simulink model "EKF_SIL_02_newdelIps"  (R2015a)
settings: Solver=ode45  StartTime=0.0  StopTime=totalSimulationTime  RelTol=1e-3
model workspace: external: MATLAB File Init_Model_02_Simulink_SIL1.m (data not in the file)
values from neighbouring files (symbols this model uses):
  Cov_nu = [0.005 0 0 0 ... (first row only)    [InitOOSM.m]    (also in InitSIL.m; Init_Model_02_Simulink.m; Init_Model_02_Simulink_SIL1.m)
  Cov_r = [0.003 0 0 ... (first row only)    [InitOOSM.m]    (also in InitSIL.m; Init_Model_02_Simulink.m; Init_Model_02_Simulink_SIL1.m)
  e_force_x = 0    [InitOOSM.m]    (also in InitSIL.m; Init_Model_02_Simulink.m; Init_Model_02_Simulink_SIL1.m)
  e_force_y = 0    [InitOOSM.m]    (also in InitSIL.m; Init_Model_02_Simulink.m; Init_Model_02_Simulink_SIL1.m)
  e_force_z = 0    [InitOOSM.m]    (also in InitSIL.m; Init_Model_02_Simulink.m; Init_Model_02_Simulink_SIL1.m)
  ieps = [-0.7071;0;0;0.7071]    [InitOOSM.m]    (also in InitSIL.m; Init_Model_02_Simulink.m = [-0.7071; 0; 0; 0.7071]; Init_Model_02_Simulink_SIL1.m)
  ita = [0.5;0.5;0.5;0.5]    [InitOOSM.m]    (also in InitSIL.m; Init_Model_02_Simulink.m = [0.5; 0.5; 0.5; 0.5]; Init_Model_02_Simulink_SIL1.m)
  n = 0.00    (= 0)    [InitOOSM.m]    (also in InitSIL.m; Init_Model_02_Simulink.m; Init_Model_02_Simulink_SIL1.m)
  P_0 = 0.5*eye(18,18)    [InitOOSM.m]    (also in InitSIL.m = 0.05*eye(12,12); Init_Model_02_Simulink.m = 0.005*eye(12,12); Init_Model_02_Simulink_SIL1.m = 0.005*eye(12,12))
  p_x = 0.75    [InitOOSM.m]    (also in InitSIL.m; Init_Model_02_Simulink.m; Init_Model_02_Simulink_SIL1.m)
  p_y = 0.125    [InitOOSM.m]    (also in InitSIL.m; Init_Model_02_Simulink.m; Init_Model_02_Simulink_SIL1.m)
  p_z = -0.8    [InitOOSM.m]    (also in InitSIL.m; Init_Model_02_Simulink.m; Init_Model_02_Simulink_SIL1.m)
  parameter_gravitation = 3.986005E+14    (= 398600500000000)    [InitOOSM.m]    (also in InitSIL.m; Init_Model_02_Simulink.m; Init_Model_02_Simulink_SIL1.m)
  rho = [0.04;0;0.3]    [InitOOSM.m]    (also in InitSIL.m; Init_Model_02_Simulink.m = [0.04; 0; 0.3]; Init_Model_02_Simulink_SIL1.m)
  rho_c = [-0.00017;   -0.9780;   -0.1854]    [InitOOSM.m]    (also in InitSIL.m = [0.00036;   -0.9865;   -0.1854]; Init_Model_02_Simulink.m = [0.00036; -0.9865; -0.1854]; Init_Model_02_Simulink_SIL1.m = [0.00036;   -0.9865;   -0.1854])
  sig_f = 2E-6    (= 2e-06)    [InitOOSM.m]    (also in InitSIL.m; Init_Model_02_Simulink.m; Init_Model_02_Simulink_SIL1.m)
  sig_tau = 2.5E-5    (= 2.5e-05)    [InitOOSM.m]    (also in InitSIL.m; Init_Model_02_Simulink.m; Init_Model_02_Simulink_SIL1.m)
  t_delta = 0.2    [InitOOSM.m]    (also in InitSIL.m; Init_Model_02_Simulink.m; Init_Model_02_Simulink_SIL1.m)
  t_Kalman = 0.01    [InitOOSM.m]    (also in InitSIL.m; Init_Model_02_Simulink.m; Init_Model_02_Simulink_SIL1.m)
  t_RobotSense = 0.05    [InitOOSM.m]    (also in InitSIL.m; Init_Model_02_Simulink.m; Init_Model_02_Simulink_SIL1.m)
  tau_1 = 0    [InitOOSM.m]    (also in InitSIL.m; Init_Model_02_Simulink.m; Init_Model_02_Simulink_SIL1.m)
  tau_2 = 0    [InitOOSM.m]    (also in InitSIL.m; Init_Model_02_Simulink.m; Init_Model_02_Simulink_SIL1.m)
  tau_3 = 0    [InitOOSM.m]    (also in InitSIL.m; Init_Model_02_Simulink.m; Init_Model_02_Simulink_SIL1.m)
  U_n_d = Simulink.Signal    [InitOOSM.m]    (also in InitSIL.m; Init_Model_02_Simulink.m; Init_Model_02_Simulink_SIL1.m)
  X_a_0 = [0; 0; 0; 1; 0; 0; 0; 0; 0; 0; 0; 0; 0;0;0;0;0;0;0;1]    [InitOOSM.m]    (also in InitSIL.m = [0; 0; 0; 1; 0; 0; 0; 0; 0; 0; 0; 0; 0]; Init_Model_02_Simulink.m = [0;0;0;0.707000000000000;0.707000000000000;0.200000000000000; Init_Model_02_Simulink_SIL1.m = [0;0;0.707;0.707;0.2;-0.02;0.0001;0.02;-1.80;0.50;-0.05;0.00)
libraries: simulink x5, dspmtrx3 x2, aerolibtransform2 x2, visionsinks x1
(part 2 of 4)

== system EKF_SIL_02_newdelIps/EKF/Measurement Update/Create X from X_a ==
  X_a(k) : Inport
  q_nominal(k) : Inport  Port=2
  ieps_nominal : Inport  Port=3
  Bus Creator1 : BusCreator  Inputs=6
  Bus Selector3 : BusSelector  OutputSignals=q_est,omega,r,r_dot,rho_c,ieps
  Bus Selector5 : BusSelector  OutputSignals=q_est,ieps
  Create Bus [State Vector,X_a] : Subsystem
  Create Bus [State Vector] : Subsystem
  Create del_q [body] : Subsystem
  Create del_q [inertial] : Subsystem
  IC : InitialCondition  Value=[X_a_0]
  X(k) : Outport
  q(k) : Outport  Port=2
  ieps(k) : Outport  Port=3
  wires:
  Create Bus [State Vector,X_a]/1(X_bus) -> Bus Selector3/1, Bus Selector5/1
  Create del_q [body]/1(del_q) -> Bus Creator1/1  "del_q"
  Bus Selector3/2 -> Bus Creator1/2  "<omega>"
  Bus Selector3/3 -> Bus Creator1/3  "<r>"
  Bus Selector3/4 -> Bus Creator1/4  "<r_dot>"
  Bus Creator1/1 -> Create Bus [State Vector]/1(X)
  Bus Selector5/1 -> Create del_q [body]/1(q)  "<q_est>"
  Create Bus [State Vector]/1(X_bus) -> X(k)/1
  X_a(k)/1 -> IC/1
  IC/1 -> Create Bus [State Vector,X_a]/1(X)
  Bus Selector3/1 -> q(k)/1  "<q_est>"
  q_nominal(k)/1 -> Create del_q [body]/2(q_nominal)
  ieps_nominal/1 -> Create del_q [inertial]/2(q_nominal)
  Bus Selector5/2 -> Create del_q [inertial]/1(q)  "<ieps>"
  Bus Selector3/5 -> Bus Creator1/5  "<rho_c>"
  Create del_q [inertial]/1(del_q) -> Bus Creator1/6  "del_ieps"
  Bus Selector3/6 -> ieps(k)/1  "<ieps>"

== system EKF_SIL_02_newdelIps/EKF/Measurement Update/Prune P ==
  P_in : Inport
  Constant : Constant  Value=2
  Divide : Product  Inputs=*/
  Math Function : Math  Operator=transpose  SaturateOnIntegerOverflow=on
  Sum : Sum  Inputs=|++
  P_out : Outport
  wires:
  P_in/1 -> Sum/2, Math Function/1
  Math Function/1 -> Sum/1
  Sum/1 -> Divide/1
  Constant/1 -> Divide/2
  Divide/1 -> P_out/1

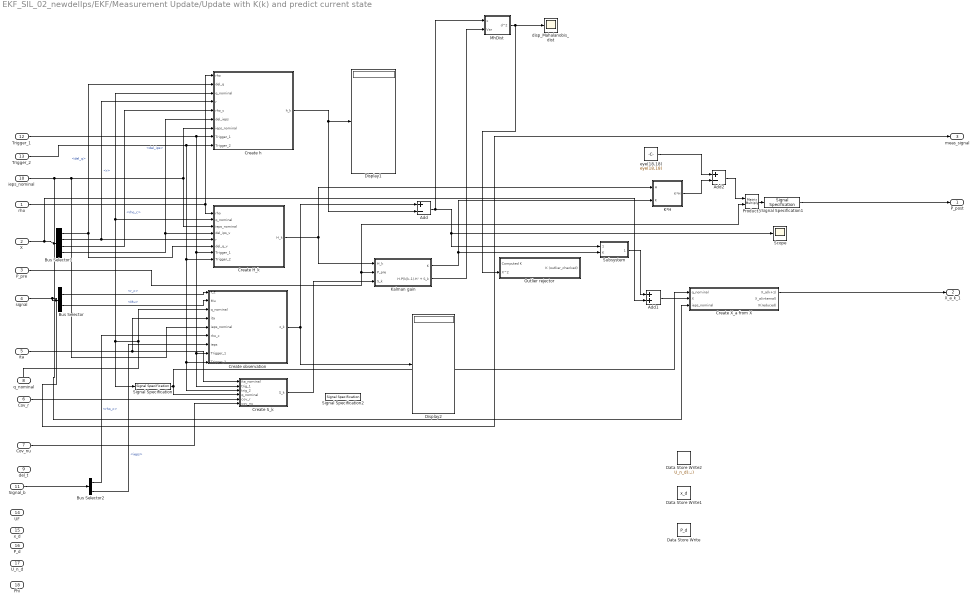
== system EKF_SIL_02_newdelIps/EKF/Measurement Update/Update with K(k) and predict current state ==
  rho : Inport
  X : Inport  Port=2
  P_pre : Inport  Port=3
  signal : Inport  Port=4
  ita : Inport  Port=5
  Cov_r : Inport  Port=6
  Cov_nu : Inport  Port=7
  q_nominal : Inport  Port=8
  del_t : Inport  Port=9
  ieps_nominal : Inport  Port=10
  Signal_b : Inport  Port=11
  Trigger_1 : Inport  Port=12
  Trigger_2 : Inport  Port=13
  UF : Inport  Port=14
  x_d : Inport  Port=15
  P_d : Inport  Port=16
  U_n_d : Inport  Port=17
  Phi : Inport  Port=18
  Add : Sum  Inputs=+-
  Add1 : Sum
  Add2 : Sum  Inputs=+-
  Bus Selector : BusSelector  OutputSignals=r_c,Mu
  Bus Selector1 : BusSelector  OutputSignals=del_q,r,rho_c,del_ips
  Bus Selector2 : BusSelector  OutputSignals=rho_c,ieps
  Create H_k : Subsystem
  Create S_k : Subsystem
  Create X_a from X : Subsystem
  Create h : Subsystem
  Create observation : Subsystem
  Data Store Write : DataStoreWrite  DataStoreName=P_d
  Data Store Write1 : DataStoreWrite  DataStoreName=x_d
  Data Store Write2 : DataStoreWrite  DataStoreName=U_n_d  DataStoreElements=U_n_d(:,:)
  Display1 : Display
  Display2 : Display
  K*H : Subsystem
  Kalman gain : Subsystem
  MhDist : Subsystem
  Outlier rejector : Subsystem
  Product3 : Product  Multiplication=Matrix(*)
  Scope : Scope
      settings: YMin=-0.005  YMax=0.03  SaveName=ScopeData10
  Signal Specification : SignalSpecification  Dimensions=[4,1]
  Signal Specification1 : SignalSpecification  Dimensions=[18,18]
  Signal Specification2 : SignalSpecification  Dimensions=[12,12]
  Subsystem : Subsystem
  disp_Mahalanobis_dist : Scope
      settings: TimeRange=100  YMin=0  YMax=32500  SaveName=ScopeData29
  eye(18,18) : Constant  Value=eye(18,18)
  P_post : Outport
  X_a_k_1 : Outport  Port=2
  meas_signal : Outport  Port=3
  wires:
  Bus Selector/1 -> Create observation/1(r_c)  "<r_c>"
  eye(18,18)/1 -> Add2/1
  Create h/1(h_k) -> Add/2, Display1/1
  Add/1 -> MhDist/1(x), Subsystem/1(residual), Scope/1
  Create observation/1(z_k) -> Add/1, Display2/1
  Bus Selector1/2 -> Create H_k/5(r), Create h/4(r)  "<r>"
  Bus Selector1/1 -> Create h/2(del_q), Create H_k/6(del_q_v)  "<del_q>"
  Create H_k/1(H_k) -> K*H/1(H), Kalman gain/1(H_k)
  P_pre/1 -> Product3/2, Kalman gain/2(P_pre)
  rho/1 -> Create h/1(rho), Create H_k/1(rho)
  Bus Selector/2 -> Create observation/2(Mu)  "<Mu>"
  Add2/1 -> Product3/1
  Signal Specification/1 -> Create S_k/4(q_nominal), Create X_a from X/1(q_nominal)
  Product3/1 -> Signal Specification1/1
  Signal Specification1/1 -> P_post/1
  ita/1 -> Create S_k/1(ita_nominal), Create observation/4(ita)
  signal/1 -> meas_signal/1, Bus Selector/1
  q_nominal/1 -> Signal Specification/1, Create h/3(q_nominal), Create H_k/2(q_nominal), Create observation/3(q_nominal)
  Create X_a from X/1(X_a(k+1)) -> X_a_k_1/1
  Kalman gain/1(K) -> Subsystem/2(K), K*H/2(K)
  Bus Selector1/3 -> Create h/5(rho_c)  "<rho_c>"
  Bus Selector1/4 -> Create h/6("del_ieps "), Create H_k/4(del_ips_v)  "<del_ips>"
  ieps_nominal/1 -> Create X_a from X/3(ieps_nominal), Create observation/5(ieps_nominal), Create H_k/3(ieps_nominal), Create h/7("ieps_nominal ")
  Add1/1 -> Create X_a from X/2(X)
  X/1 -> Add1/2, Bus Selector1/1
  Signal_b/1 -> Bus Selector2/1
  Bus Selector2/1 -> Create observation/6(rho_c)  "<rho_c>"
  Bus Selector2/2 -> Create observation/7(ieps)  "<ieps>"
  Trigger_1/1 -> Create h/8(Trigger_1), Create H_k/7(Trigger_1), Create S_k/2(trig_1), Create observation/8(Trigger_1)
  Trigger_2/1 -> Create h/9(Trigger_2), Create H_k/8(Trigger_2), Create observation/9(Trigger_2), Create S_k/3(trig_2)
  Cov_r/1 -> Create S_k/5(cov_r)
  Cov_nu/1 -> Create S_k/6(cov_nu)
  Create S_k/1(S_k) -> Kalman gain/3(S_k)
  K*H/1(K*H) -> Add2/2
  Subsystem/1(K(z-h(x))) -> Add1/1
  MhDist/1(d^2) -> Outlier rejector/2(X^2), disp_Mahalanobis_dist/1
  Kalman gain/2(H.P(k|k-1).H' + S_k) -> MhDist/2(Var)

== system EKF_SIL_02_newdelIps/EKF/Predictor/Create Bus [State Vector,X_a] ==
  X : Inport
  Bus Creator{1,3..5} (4 alike) : BusCreator  Inputs=3
  Bus Creator2 : BusCreator
  Bus Creator6 : BusCreator  Inputs=6
  Bus Creator7 : BusCreator
  Demux1 : Demux  Outputs=20
  X_bus : Outport
  wires:
  Bus Creator2/1 -> Bus Creator6/1  "q_est"
  Bus Creator3/1 -> Bus Creator6/2  "omega"
  Bus Creator4/1 -> Bus Creator6/3  "r"
  Bus Creator5/1 -> Bus Creator6/4  "r_dot"
  Bus Creator6/1 -> X_bus/1
  X/1 -> Demux1/1
  Demux1/1 -> Bus Creator2/1  "q_est_1"
  Demux1/2 -> Bus Creator2/2  "q_est_2"
  Demux1/3 -> Bus Creator2/3  "q_est_3"
  Demux1/4 -> Bus Creator2/4  "q_est_0"
  Demux1/5 -> Bus Creator3/1  "omega_x"
  Demux1/6 -> Bus Creator3/2  "omega_y"
  Demux1/7 -> Bus Creator3/3  "omega_z"
  Demux1/8 -> Bus Creator4/1  "r_x"
  Demux1/9 -> Bus Creator4/2  "r_y"
  Demux1/10 -> Bus Creator4/3  "r_z"
  Demux1/11 -> Bus Creator5/1  "r_x_dot"
  Demux1/12 -> Bus Creator5/2  "r_y_dot"
  Demux1/13 -> Bus Creator5/3  "r_z_dot"
  Demux1/14 -> Bus Creator1/1  "rho_c_x"
  Demux1/15 -> Bus Creator1/2  "rho_c_y"
  Demux1/16 -> Bus Creator1/3  "rho_c_z"
  Demux1/17 -> Bus Creator7/1  "ieps_1"
  Demux1/18 -> Bus Creator7/2  "ieps_2"
  Demux1/19 -> Bus Creator7/3  "ieps_3"
  Demux1/20 -> Bus Creator7/4  "ieps_0"
  Bus Creator1/1 -> Bus Creator6/5  "rho_c"
  Bus Creator7/1 -> Bus Creator6/6  "ieps"

== system EKF_SIL_02_newdelIps/EKF/Predictor/Create Bus [State Vector,X_a]1 ==
  X : Inport
  Bus Creator{1,3..5} (4 alike) : BusCreator  Inputs=3
  Bus Creator2 : BusCreator
  Bus Creator6 : BusCreator  Inputs=6
  Bus Creator7 : BusCreator
  Demux1 : Demux  Outputs=20
  X_bus : Outport
  wires:
  Bus Creator2/1 -> Bus Creator6/1  "q_est"
  Bus Creator3/1 -> Bus Creator6/2  "omega"
  Bus Creator4/1 -> Bus Creator6/3  "r"
  Bus Creator5/1 -> Bus Creator6/4  "r_dot"
  Bus Creator6/1 -> X_bus/1
  X/1 -> Demux1/1
  Demux1/1 -> Bus Creator2/1  "q_est_1"
  Demux1/2 -> Bus Creator2/2  "q_est_2"
  Demux1/3 -> Bus Creator2/3  "q_est_3"
  Demux1/4 -> Bus Creator2/4  "q_est_0"
  Demux1/5 -> Bus Creator3/1  "omega_x"
  Demux1/6 -> Bus Creator3/2  "omega_y"
  Demux1/7 -> Bus Creator3/3  "omega_z"
  Demux1/8 -> Bus Creator4/1  "r_x"
  Demux1/9 -> Bus Creator4/2  "r_y"
  Demux1/10 -> Bus Creator4/3  "r_z"
  Demux1/11 -> Bus Creator5/1  "r_x_dot"
  Demux1/12 -> Bus Creator5/2  "r_y_dot"
  Demux1/13 -> Bus Creator5/3  "r_z_dot"
  Demux1/14 -> Bus Creator1/1  "rho_c_x"
  Demux1/15 -> Bus Creator1/2  "rho_c_y"
  Demux1/16 -> Bus Creator1/3  "rho_c_z"
  Demux1/17 -> Bus Creator7/1  "ieps_1"
  Demux1/18 -> Bus Creator7/2  "ieps_2"
  Demux1/19 -> Bus Creator7/3  "ieps_3"
  Demux1/20 -> Bus Creator7/4  "ieps_0"
  Bus Creator1/1 -> Bus Creator6/5  "rho_c"
  Bus Creator7/1 -> Bus Creator6/6  "ieps"

== system EKF_SIL_02_newdelIps/EKF/Predictor/Create State error covariance (P) ==
  X_a : Inport
  P_previous : Inport  Port=2
  V : Inport  Port=3
  Add : Sum
  Math Function : Math  Operator=transpose  SaturateOnIntegerOverflow=on
  Matrix Concatenate : Concatenate  NumInputs=3  Mode=Multidimensional array  ConcatenateDimension=2
  Matrix Concatenate1 : Concatenate  NumInputs=3  Mode=Multidimensional array
  Matrix Concatenate2 : Concatenate  NumInputs=3  Mode=Multidimensional array  ConcatenateDimension=2
  Matrix Concatenate3 : Concatenate  NumInputs=3  Mode=Multidimensional array  ConcatenateDimension=2
  "Process Noise [Robot motion] " : Constant  Value=1e-15*eye(6,6)
  Process noise covariance [rotational] : Subsystem
  Process noise covariance [translational] : Subsystem
  Product : Product  Inputs=3  Multiplication=Matrix(*)
  State Propagation : Subsystem
  zeros(6,6) : Constant  Value=zeros(6,6)
  P_current : Outport
  wires:
  Math Function/1 -> Product/3
  P_previous/1 -> Product/2
  Add/1 -> P_current/1
  X_a/1 -> State Propagation/1("X_a(t)\t")
  Product/1 -> Add/2
  Matrix Concatenate2/1 -> Matrix Concatenate1/2
  Matrix Concatenate/1 -> Matrix Concatenate1/1
  zeros(6,6)/1 -> Matrix Concatenate/3, Matrix Concatenate/2, Matrix Concatenate2/3, Matrix Concatenate3/2, Matrix Concatenate3/1, Matrix Concatenate2/1
  State Propagation/1(Phi) -> Math Function/1, Product/1, Process noise covariance [rotational]/1(Phi)
  V/1 -> State Propagation/2(V)
  "Process Noise [Robot motion] "/1 -> Matrix Concatenate3/3
  Matrix Concatenate3/1 -> Matrix Concatenate1/3
  Matrix Concatenate1/1 -> Add/1
  Process noise covariance [rotational]/1(Q_r) -> Matrix Concatenate/1
  Process noise covariance [translational]/1(Q_t) -> Matrix Concatenate2/2

== system EKF_SIL_02_newdelIps/EKF/Predictor/Dynamic Model (Differential equations)2 ==
  X_a(t) : Inport
  "V " : Inport  Port=2
  Dynamic Model (Differential equations) : Subsystem
  X_a_dot : Outport
  wires:
  X_a(t)/1 -> Dynamic Model (Differential equations)/1(X_a(t))
  Dynamic Model (Differential equations)/1(X_a(t+1)) -> X_a_dot/1
  "V "/1 -> Dynamic Model (Differential equations)/2("V ")

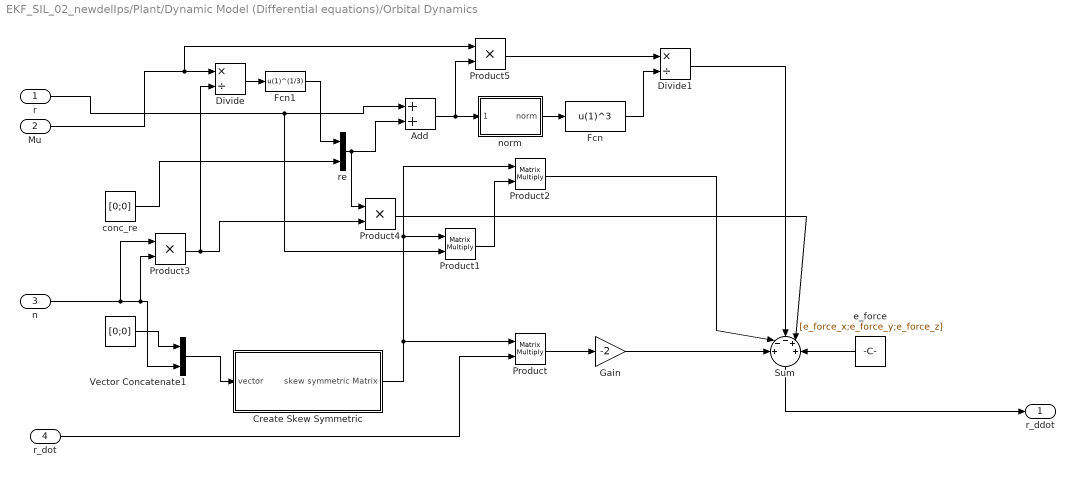
== system EKF_SIL_02_newdelIps/Plant/Dynamic Model (Differential equations)/Orbital Dynamics  ==
  r : Inport
  Mu : Inport  Port=2
  n : Inport  Port=3
  "r_dot " : Inport  Port=4
  " " : Constant  Value=[0;0]
  Add : Sum
  Create Skew Symmetric : Subsystem
  Divide : Product  Inputs=*/
  Divide1 : Product  Inputs=*/
  Fcn : Fcn  Expr=u(1)^3
  Fcn1 : Fcn  Expr=u(1)^(1/3)
  Gain : Gain  Gain=-2
  Product : Product  Multiplication=Matrix(*)
  Product1 : Product  Multiplication=Matrix(*)
  Product2 : Product  Multiplication=Matrix(*)
  Product3 : Product
  Product4 : Product
  Product5 : Product
  Sum : Sum  Inputs=+--++
  Vector Concatenate1 : Concatenate
  "conc_re " : Constant  Value=[0;0]
  "e_force " : Constant  Value=[e_force_x;e_force_y;e_force_z]
  "norm " : Subsystem
  re : Concatenate
  "r_ddot " : Outport
  wires:
  " "/1 -> Vector Concatenate1/1
  Create Skew Symmetric/1(skew symmetric Matrix) -> Product/1, Product1/1, Product2/1
  Product1/1 -> Product2/2
  Mu/1 -> Product5/1, Divide/1
  Product/1 -> Gain/1
  "conc_re "/1 -> re/2
  re/1 -> Product4/1, Add/2
  Product5/1 -> Divide1/1
  "norm "/1("norm ") -> Fcn/1
  n/1 -> Product3/2, Vector Concatenate1/2, Product3/1
  Product3/1 -> Divide/2, Product4/2
  Vector Concatenate1/1 -> Create Skew Symmetric/1(vector)
  Add/1 -> "norm "/1(vector), Product5/2
  Gain/1 -> Sum/1
  Product2/1 -> Sum/2
  r/1 -> Product1/2, Add/1
  Product4/1 -> Sum/4
  "r_dot "/1 -> Product/2
  Divide1/1 -> Sum/3
  Fcn1/1 -> re/1
  Fcn/1 -> Divide1/2
  Divide/1 -> Fcn1/1
  "e_force "/1 -> Sum/5
  Sum/1 -> "r_ddot "/1

== system EKF_SIL_02_newdelIps/Plant/Dynamic Model (Differential equations)/Quaternion Kinematics ==
  q : Inport
  omega_rel : Inport  Port=2
  Constant2 : Constant  Value=0.5
  MATLAB Function : MATLAB Function  TreatAsAtomicUnit=on
  Product : Product  Multiplication=Matrix(*)
  Product1 : Product
  flag : Constant
  q_dot : Outport
  wires:
  MATLAB Function/1(CrossTensor) -> Product/1
  flag/1 -> MATLAB Function/2(flag)
  Constant2/1 -> Product1/2
  q/1 -> MATLAB Function/1(q)
  omega_rel/1 -> Product/2
  Product1/1 -> q_dot/1
  Product/1 -> Product1/1

== system EKF_SIL_02_newdelIps/Plant/Dynamic Model (Differential equations)/Rotational Dynamics ==
  omega : Inport
  p : Inport  Port=2
  Add : Sum
  Create  J : Subsystem
  Create Psi : Subsystem
  Product : Product  Multiplication=Matrix(*)
  tau : Constant  Value=[tau_1;tau_2;tau_3]
  omega_dot : Outport
  wires:
  omega/1 -> Create Psi/1("omega ")
  Create Psi/1(Psi) -> Add/1
  Add/1 -> omega_dot/1
  Product/1 -> Add/2
  p/1 -> Create Psi/2(p), Create  J/1(p)
  Create  J/1("J_k ") -> Product/1
  tau/1 -> Product/2

== system EKF_SIL_02_newdelIps/Plots and display/Create Measurements [Pose]1/Create Measurements [Orientation]  ==
  q : Inport
  "ita " : Inport  Port=2
  Bus Creator : BusCreator
  Demux : Demux
  MATLAB Function : MATLAB Function  TreatAsAtomicUnit=on
  Product : Product  Multiplication=Matrix(*)
  "flag " : Constant  Value=0
  Mu : Outport
  wires:
  Product/1 -> Demux/1
  q/1 -> Product/2
  Bus Creator/1 -> Mu/1  "Mu"
  "ita "/1 -> MATLAB Function/1(q)
  MATLAB Function/1(CrossTensor) -> Product/1
  "flag "/1 -> MATLAB Function/2(flag)
  Demux/1 -> Bus Creator/1
  Demux/2 -> Bus Creator/2
  Demux/3 -> Bus Creator/3
  Demux/4 -> Bus Creator/4

== system EKF_SIL_02_newdelIps/Plots and display/Create Measurements [Pose]1/Create Measurements [Position] ==
  r : Inport
  q : Inport  Port=2
  rho : Inport  Port=3
  "rho_c " : Inport  Port=4
  Add : Sum  Inputs=+++
  Bus Creator : BusCreator  Inputs=3
  "Create Rotation Matrix " : Subsystem
  Demux : Demux  Outputs=3
  Product : Product  Multiplication=Matrix(*)
  r_c : Outport
  wires:
  Add/1 -> Demux/1
  r/1 -> Add/2
  Bus Creator/1 -> r_c/1  "r_c"
  q/1 -> "Create Rotation Matrix "/1(q)
  "rho_c "/1 -> Add/1
  rho/1 -> Product/2
  "Create Rotation Matrix "/1(R) -> Product/1
  Product/1 -> Add/3
  Demux/1 -> Bus Creator/1  "r_c_x"
  Demux/2 -> Bus Creator/2  "r_c_y"
  Demux/3 -> Bus Creator/3  "r_c_z"

== system EKF_SIL_02_newdelIps/Plots and display/Create Measurements [Pose]2/Create Measurements [Orientation]  ==
  q : Inport
  "ita " : Inport  Port=2
  "ieps " : Inport  Port=3
  Bus Creator : BusCreator
  Demux : Demux
  MATLAB Function : MATLAB Function  TreatAsAtomicUnit=on
  MATLAB Function1 : MATLAB Function  TreatAsAtomicUnit=on
  Product : Product  Multiplication=Matrix(*)
  Product1 : Product  Multiplication=Matrix(*)
  "flag " : Constant  Value=0
  Mu : Outport
  wires:
  Demux/4 -> Bus Creator/4
  Demux/3 -> Bus Creator/3
  Demux/2 -> Bus Creator/2
  Demux/1 -> Bus Creator/1
  "flag "/1 -> MATLAB Function1/2(flag), MATLAB Function/2(flag)
  MATLAB Function/1(CrossTensor) -> Product/1
  "ita "/1 -> MATLAB Function/1(q)
  Bus Creator/1 -> Mu/1  "Mu"
  q/1 -> Product/2
  Product/1 -> MATLAB Function1/1(q)
  MATLAB Function1/1(CrossTensor) -> Product1/1
  "ieps "/1 -> Product1/2
  Product1/1 -> Demux/1

== system EKF_SIL_02_newdelIps/Plots and display/Create Measurements [Pose]2/Create Measurements [Position] ==
  r : Inport
  q : Inport  Port=2
  rho : Inport  Port=3
  "rho_c " : Inport  Port=4
  "ieps " : Inport  Port=5
  Add : Sum
  Add1 : Sum
  Bus Creator : BusCreator  Inputs=3
  "Create Rotation Matrix " : Subsystem
  Create Rotation Matrix 1 : Subsystem
  Demux : Demux  Outputs=3
  Product : Product  Multiplication=Matrix(*)
  Product1 : Product  Multiplication=Matrix(*)
  r_c : Outport
  wires:
  Demux/3 -> Bus Creator/3  "r_c_z"
  Demux/2 -> Bus Creator/2  "r_c_y"
  Demux/1 -> Bus Creator/1  "r_c_x"
  Product/1 -> Add/2
  "Create Rotation Matrix "/1(R) -> Product/1
  rho/1 -> Product/2
  q/1 -> "Create Rotation Matrix "/1(q)
  Bus Creator/1 -> r_c/1  "r_c"
  r/1 -> Add/1
  Create Rotation Matrix 1/1(R) -> Product1/1
  "rho_c "/1 -> Add1/2
  Add1/1 -> Demux/1
  Add/1 -> Product1/2
  "ieps "/1 -> Create Rotation Matrix 1/1(q)
  Product1/1 -> Add1/1

== system EKF_SIL_02_newdelIps/EKF/Measurement Update/Create X from X_a/Create Bus [State Vector,X_a] ==
  X : Inport
  Bus Creator{1,3..5} (4 alike) : BusCreator  Inputs=3
  Bus Creator2 : BusCreator
  Bus Creator6 : BusCreator  Inputs=6
  Bus Creator7 : BusCreator
  Demux1 : Demux  Outputs=20
  X_bus : Outport
  wires:
  Bus Creator2/1 -> Bus Creator6/1  "q_est"
  Bus Creator3/1 -> Bus Creator6/2  "omega"
  Bus Creator4/1 -> Bus Creator6/3  "r"
  Bus Creator5/1 -> Bus Creator6/4  "r_dot"
  Bus Creator6/1 -> X_bus/1
  X/1 -> Demux1/1
  Demux1/1 -> Bus Creator2/1  "q_est_1"
  Demux1/2 -> Bus Creator2/2  "q_est_2"
  Demux1/3 -> Bus Creator2/3  "q_est_3"
  Demux1/4 -> Bus Creator2/4  "q_est_0"
  Demux1/5 -> Bus Creator3/1  "omega_x"
  Demux1/6 -> Bus Creator3/2  "omega_y"
  Demux1/7 -> Bus Creator3/3  "omega_z"
  Demux1/8 -> Bus Creator4/1  "r_x"
  Demux1/9 -> Bus Creator4/2  "r_y"
  Demux1/10 -> Bus Creator4/3  "r_z"
  Demux1/11 -> Bus Creator5/1  "r_x_dot"
  Demux1/12 -> Bus Creator5/2  "r_y_dot"
  Demux1/13 -> Bus Creator5/3  "r_z_dot"
  Demux1/14 -> Bus Creator1/1  "rho_c_x"
  Demux1/15 -> Bus Creator1/2  "rho_c_y"
  Demux1/16 -> Bus Creator1/3  "rho_c_z"
  Demux1/17 -> Bus Creator7/1  "ieps_1"
  Demux1/18 -> Bus Creator7/2  "ieps_2"
  Demux1/19 -> Bus Creator7/3  "ieps_3"
  Demux1/20 -> Bus Creator7/4  "ieps_0"
  Bus Creator1/1 -> Bus Creator6/5  "rho_c"
  Bus Creator7/1 -> Bus Creator6/6  "ieps"

== system EKF_SIL_02_newdelIps/EKF/Measurement Update/Create X from X_a/Create Bus [State Vector] ==
  X : Inport
  Bus Creator{1..5,7} (6 alike) : BusCreator  Inputs=3
  Bus Creator6 : BusCreator  Inputs=6
  Demux1 : Demux  Outputs=18
  X_bus : Outport
  wires:
  Demux1/4 -> Bus Creator3/1  "omega_x"
  Bus Creator2/1 -> Bus Creator6/1  "del_q"
  Demux1/8 -> Bus Creator4/2  "r_y"
  Demux1/6 -> Bus Creator3/3  "omega_z"
  Demux1/7 -> Bus Creator4/1  "r_x"
  Demux1/10 -> Bus Creator5/1  "r_x_dot"
  Bus Creator3/1 -> Bus Creator6/2  "omega"
  Demux1/3 -> Bus Creator2/3  "del_q_3"
  Demux1/1 -> Bus Creator2/1  "del_q_1"
  Demux1/11 -> Bus Creator5/2  "r_y_dot"
  Demux1/12 -> Bus Creator5/3  "r_z_dot"
  Demux1/2 -> Bus Creator2/2  "del_q_2"
  Demux1/5 -> Bus Creator3/2  "omega_y"
  Demux1/9 -> Bus Creator4/3  "r_z"
  Bus Creator4/1 -> Bus Creator6/3  "r"
  Bus Creator5/1 -> Bus Creator6/4  "r_dot"
  Bus Creator6/1 -> X_bus/1
  X/1 -> Demux1/1
  Demux1/13 -> Bus Creator1/1  "rho_c_x"
  Demux1/14 -> Bus Creator1/2  "rho_c_y"
  Demux1/15 -> Bus Creator1/3  "rho_c_z"
  Demux1/16 -> Bus Creator7/1  "del_ieps_1"
  Demux1/17 -> Bus Creator7/2
  Demux1/18 -> Bus Creator7/3  "del_ips_3"
  Bus Creator1/1 -> Bus Creator6/5  "rho_c"
  Bus Creator7/1 -> Bus Creator6/6  "del_ips"

== system EKF_SIL_02_newdelIps/EKF/Measurement Update/Create X from X_a/Create del_q [body] ==
  q : Inport
  q_nominal : Inport  Port=2
  Constant : Constant  Value=0
  Demux : Demux
  MATLAB Function : MATLAB Function  TreatAsAtomicUnit=on
  Mux : Mux  Inputs=3
  Product : Product  Multiplication=Matrix(*)
  Scope : Scope
      settings: SaveName=ScopeData6
  q_star : Subsystem
  del_q : Outport
  wires:
  q_star/1(q_star) -> Product/2
  MATLAB Function/1(CrossTensor) -> Product/1
  q/1 -> MATLAB Function/1(q)
  Constant/1 -> MATLAB Function/2(flag)
  q_nominal/1 -> q_star/1(q)
  Product/1 -> Demux/1
  Demux/1 -> Mux/1
  Demux/2 -> Mux/2
  Demux/3 -> Mux/3
  Mux/1 -> del_q/1
  Demux/4 -> Scope/1

== system EKF_SIL_02_newdelIps/EKF/Measurement Update/Create X from X_a/Create del_q [inertial] ==
  q : Inport
  q_nominal : Inport  Port=2
  Constant : Constant  Value=0
  Demux : Demux
  MATLAB Function : MATLAB Function  TreatAsAtomicUnit=on
  Mux : Mux  Inputs=3
  Product : Product  Multiplication=Matrix(*)
  Scope : Scope
      settings: SaveName=ScopeData6
  q_star : Subsystem
  del_q : Outport
  wires:
  q_star/1(q_star) -> Product/2
  MATLAB Function/1(CrossTensor) -> Product/1
  q/1 -> MATLAB Function/1(q)
  Constant/1 -> MATLAB Function/2(flag)
  q_nominal/1 -> q_star/1(q)
  Product/1 -> Demux/1
  Demux/1 -> Mux/1
  Demux/2 -> Mux/2
  Demux/3 -> Mux/3
  Mux/1 -> del_q/1
  Demux/4 -> Scope/1

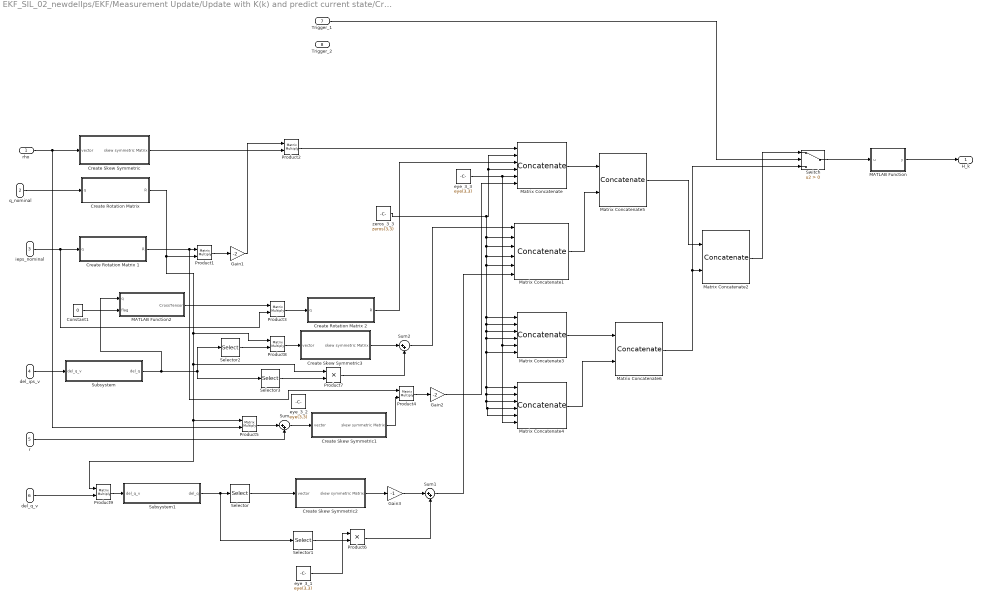
== system EKF_SIL_02_newdelIps/EKF/Measurement Update/Update with K(k) and predict current state/Create H_k ==
  rho : Inport
  q_nominal : Inport  Port=2
  ieps_nominal : Inport  Port=3
  del_ips_v : Inport  Port=4
  r : Inport  Port=5
  del_q_v : Inport  Port=6
  Trigger_1 : Inport  Port=7
  Trigger_2 : Inport  Port=8
  Constant1 : Constant  Value=0
  "Create Rotation Matrix " : Subsystem
  Create Rotation Matrix 1 : Subsystem
  Create Rotation Matrix 2 : Subsystem
  Create Skew Symmetric : Subsystem
  Create Skew Symmetric1 : Subsystem
  Create Skew Symmetric2 : Subsystem
  Create Skew Symmetric3 : Subsystem
  Gain1 : Gain  Gain=-2
  Gain2 : Gain  Gain=-2
  Gain3 : Gain  Gain=-1
  MATLAB Function : MATLAB Function  TreatAsAtomicUnit=on
  MATLAB Function2 : MATLAB Function  TreatAsAtomicUnit=on
  Matrix Concatenate{,1,3..4} (4 alike) : Concatenate  NumInputs=6  Mode=Multidimensional array  ConcatenateDimension=2
  Matrix Concatenate2 : Concatenate  Mode=Multidimensional array
  Matrix Concatenate5 : Concatenate  Mode=Multidimensional array
  Matrix Concatenate6 : Concatenate  Mode=Multidimensional array
  Product{1..5,8..9} (7 alike) : Product  Multiplication=Matrix(*)
  Product6 : Product
  Product7 : Product
  Selector : Selector  InputPortWidth=4  Indices=[1:3]
  Selector1 : Selector  InputPortWidth=4  Indices=4
  Selector2 : Selector  InputPortWidth=4  Indices=[1:3]
  Selector3 : Selector  InputPortWidth=4  Indices=4
  Subsystem : Subsystem
  Subsystem1 : Subsystem
  Sum : Sum  Inputs=|++
  Sum1 : Sum  Inputs=|++
  Sum2 : Sum  Inputs=|++
  Switch : Switch  Criteria=u2 > Threshold  AllowDiffInputSizes=on
  eye_3_1 : Constant  Value=eye(3,3)
  eye_3_2 : Constant  Value=eye(3,3)
  eye_3_3 : Constant  Value=eye(3,3)
  zeros_3_3 : Constant  Value=zeros(3,3)
  H_k : Outport
  wires:
  q_nominal/1 -> "Create Rotation Matrix "/1(q)
  Switch/1 -> MATLAB Function/1(u)
  eye_3_3/1 -> Matrix Concatenate4/6, Matrix Concatenate3/5, Matrix Concatenate/5
  Create Skew Symmetric/1(skew symmetric Matrix) -> Product2/2
  rho/1 -> Product5/2, Create Skew Symmetric/1(vector)
  Create Rotation Matrix 1/1(R) -> Product4/1, Product1/1
  Product1/1 -> Gain1/1
  Gain1/1 -> Product2/1
  Product2/1 -> Matrix Concatenate/1
  del_ips_v/1 -> Subsystem/1(del_q_v)
  Constant1/1 -> MATLAB Function2/2(flag)
  MATLAB Function2/1(CrossTensor) -> Product3/1
  ieps_nominal/1 -> Product3/2, Create Rotation Matrix 1/1(q)
  Create Rotation Matrix 2/1(R) -> Matrix Concatenate/3
  "Create Rotation Matrix "/1(R) -> Product7/1, Product9/1, Product5/1, Product8/1, Product1/2
  Product5/1 -> Sum/1
  r/1 -> Sum/2
  Gain2/1 -> Matrix Concatenate/6
  Subsystem1/1(del_q) -> Selector1/1, Selector/1
  Selector/1 -> Create Skew Symmetric2/1(vector)
  Create Skew Symmetric2/1(skew symmetric Matrix) -> Gain3/1
  Selector1/1 -> Product6/2
  eye_3_1/1 -> Product6/1
  Gain3/1 -> Sum1/1
  Product6/1 -> Sum1/2
  Sum1/1 -> Matrix Concatenate1/6
  Selector2/1 -> Product8/2
  Create Skew Symmetric3/1(skew symmetric Matrix) -> Sum2/1
  Selector3/1 -> Product7/2
  Product7/1 -> Sum2/2
  Sum2/1 -> Matrix Concatenate1/1
  Sum/1 -> Create Skew Symmetric1/1(vector)
  Create Skew Symmetric1/1(skew symmetric Matrix) -> Product4/2
  Product3/1 -> Create Rotation Matrix 2/1(q)
  zeros_3_3/1 -> Matrix Concatenate3/6, Matrix Concatenate4/1, Matrix Concatenate4/5, Matrix Concatenate4/4, Matrix Concatenate4/3, Matrix Concatenate4/2, Matrix Concatenate3/4, Matrix Concatenate3/3, Matrix Concatenate3/2, Matrix Concatenate3/1, Matrix Concatenate1/5, Matrix Concatenate1/4, Matrix Concatenate1/3, Matrix Concatenate1/2, Matrix Concatenate/4, Matrix Concatenate/2
  Matrix Concatenate1/1 -> Matrix Concatenate5/2
  Matrix Concatenate4/1 -> Matrix Concatenate6/2
  Subsystem/1(del_q) -> MATLAB Function2/1(q), Selector2/1, Selector3/1
  del_q_v/1 -> Product9/2
  Product9/1 -> Subsystem1/1(del_q_v)
  Product8/1 -> Create Skew Symmetric3/1(vector)
  Product4/1 -> Gain2/1
  Matrix Concatenate/1 -> Matrix Concatenate5/1
  Matrix Concatenate3/1 -> Matrix Concatenate6/1
  Trigger_1/1 -> Switch/2
  Matrix Concatenate5/1 -> Matrix Concatenate2/1
  Matrix Concatenate6/1 -> Switch/3, Matrix Concatenate2/2
  Matrix Concatenate2/1 -> Switch/1
  MATLAB Function/1(y) -> H_k/1

== system EKF_SIL_02_newdelIps/EKF/Measurement Update/Update with K(k) and predict current state/Create S_k ==
  ita_nominal : Inport
  trig_1 : Inport  Port=2
  trig_2 : Inport  Port=3
  q_nominal : Inport  Port=4
  cov_r : Inport  Port=5
  cov_nu : Inport  Port=6
  Constant : Constant  Value=1e-5*eye(6,6)
  Constant1 : Constant  Value=zeros(6,6)
  Matrix Concatenate1 : Concatenate  Mode=Multidimensional array
  Matrix Concatenate5 : Concatenate  Mode=Multidimensional array  ConcatenateDimension=2
  Matrix Concatenate6 : Concatenate  Mode=Multidimensional array  ConcatenateDimension=2
  Measurement noise covariance : MATLAB Function  TreatAsAtomicUnit=on
  Switch : Switch  Criteria=u2 > Threshold  AllowDiffInputSizes=on
  S_k : Outport
  wires:
  q_nominal/1 -> Measurement noise covariance/1(q_nominal)
  ita_nominal/1 -> Measurement noise covariance/2(ita_nominal)
  cov_nu/1 -> Measurement noise covariance/4(cov_nu)
  cov_r/1 -> Measurement noise covariance/3(cov_r)
  Measurement noise covariance/1(S) -> Matrix Concatenate5/1, Switch/3
  trig_1/1 -> Switch/2
  Constant1/1 -> Matrix Concatenate6/1, Matrix Concatenate5/2
  Constant/1 -> Matrix Concatenate6/2
  Switch/1 -> S_k/1
  Matrix Concatenate1/1 -> Switch/1
  Matrix Concatenate5/1 -> Matrix Concatenate1/1
  Matrix Concatenate6/1 -> Matrix Concatenate1/2

== system EKF_SIL_02_newdelIps/EKF/Measurement Update/Update with K(k) and predict current state/Create X_a from X ==
  q_nominal : Inport
  X : Inport  Port=2
  ieps_nominal : Inport  Port=3
  Bus Creator1 : BusCreator
  Bus Creator2 : BusCreator  Inputs=6
  Bus Creator3 : BusCreator
  Bus Selector2 : BusSelector  OutputSignals=del_q,del_ips
  Bus Selector3 : BusSelector  OutputSignals=omega,r,r_dot,rho_c
  Create Bus [State Vector] : Subsystem
  "Create ieps " : Subsystem
  "Create q_nominal " : Subsystem
  Demux : Demux
  Demux1 : Demux
  Display2 : Display
  Signal Conversion : SignalConversion
  X_a(k+1) : Outport
  X_a(internal) : Outport  Port=2
  "X(reduced) " : Outport  Port=3
  wires:
  Bus Selector3/3 -> Bus Creator2/4  "<r_dot>"
  Demux/1 -> Bus Creator3/1  "q_est_1"
  Bus Selector3/2 -> Bus Creator2/3  "<r>"
  Bus Creator3/1 -> Bus Creator2/1  "q_est"
  Create Bus [State Vector]/1(X_bus) -> "X(reduced) "/1, Bus Selector3/1, Bus Selector2/1
  X/1 -> Create Bus [State Vector]/1(X)
  Bus Selector3/1 -> Bus Creator2/2  "<omega>"
  Demux/2 -> Bus Creator3/2  "q_est_2"
  Demux/4 -> Bus Creator3/4  "q_est_0"
  Demux/3 -> Bus Creator3/3  "q_est_3"
  Bus Creator2/1 -> X_a(internal)/1, Signal Conversion/1
  Bus Selector2/1 -> "Create q_nominal "/1(del_q)  "<del_q>"
  q_nominal/1 -> "Create q_nominal "/2(q_nominal)
  "Create q_nominal "/1(q_est) -> Demux/1
  Signal Conversion/1 -> X_a(k+1)/1
  Bus Selector2/2 -> "Create ieps "/1(del_q)  "<del_ips>"
  ieps_nominal/1 -> "Create ieps "/2(q_nominal)
  Bus Selector3/4 -> Bus Creator2/5  "<rho_c>"
  Demux1/1 -> Bus Creator1/1  "ieps_est_1"
  Bus Creator1/1 -> Bus Creator2/6  "ieps_est"
  Demux1/2 -> Bus Creator1/2  "ieps_est_2"
  Demux1/4 -> Bus Creator1/4  "ieps_est_0"
  Demux1/3 -> Bus Creator1/3  "ieps_est_3"
  "Create ieps "/1(q_est) -> Display2/1, Demux1/1

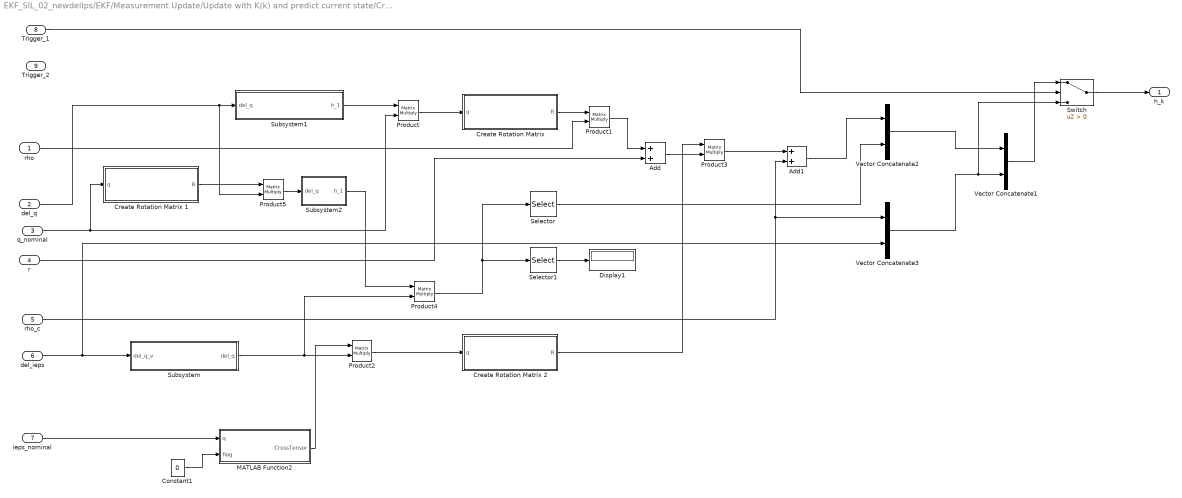
== system EKF_SIL_02_newdelIps/EKF/Measurement Update/Update with K(k) and predict current state/Create h ==
  rho : Inport
  del_q : Inport  Port=2
  q_nominal : Inport  Port=3
  r : Inport  Port=4
  rho_c : Inport  Port=5
  "del_ieps " : Inport  Port=6
  "ieps_nominal " : Inport  Port=7
  Trigger_1 : Inport  Port=8
  Trigger_2 : Inport  Port=9
  Add : Sum
  Add1 : Sum
  Constant1 : Constant  Value=0
  "Create Rotation Matrix " : Subsystem
  Create Rotation Matrix 1 : Subsystem
  Create Rotation Matrix 2 : Subsystem
  Display1 : Display
  MATLAB Function2 : MATLAB Function  TreatAsAtomicUnit=on
  Product{,1..5} (6 alike) : Product  Multiplication=Matrix(*)
  Selector : Selector  InputPortWidth=4  Indices=[1:3]
  Selector1 : Selector  InputPortWidth=4  Indices=4
  Subsystem : Subsystem
  Subsystem1 : Subsystem
  Subsystem2 : Subsystem
  Switch : Switch  Criteria=u2 > Threshold  AllowDiffInputSizes=on
  Vector Concatenate1 : Concatenate
  Vector Concatenate2 : Concatenate
  Vector Concatenate3 : Concatenate
  h_k : Outport
  wires:
  rho/1 -> Product1/2
  q_nominal/1 -> Product/2, Create Rotation Matrix 1/1(q)
  "Create Rotation Matrix "/1(R) -> Product1/1
  del_q/1 -> Product5/2, Subsystem1/1(del_q)
  Product/1 -> "Create Rotation Matrix "/1(q)
  Subsystem1/1(h_1) -> Product/1
  Product1/1 -> Add/1
  rho_c/1 -> Vector Concatenate3/1, Add1/2
  "del_ieps "/1 -> Vector Concatenate3/2, Subsystem/1(del_q_v)
  "ieps_nominal "/1 -> MATLAB Function2/1(q)
  Constant1/1 -> MATLAB Function2/2(flag)
  Subsystem/1(del_q) -> Product4/2, Product2/2
  MATLAB Function2/1(CrossTensor) -> Product2/1
  Product2/1 -> Create Rotation Matrix 2/1(q)
  Create Rotation Matrix 2/1(R) -> Product3/1
  Product3/1 -> Add1/1
  Add/1 -> Product3/2
  Add1/1 -> Vector Concatenate2/1
  Product4/1 -> Selector1/1, Selector/1
  r/1 -> Add/2
  Selector1/1 -> Display1/1
  Create Rotation Matrix 1/1(R) -> Product5/1
  Product5/1 -> Subsystem2/1(del_q)
  Subsystem2/1(h_1) -> Product4/1
  Selector/1 -> Vector Concatenate2/2
  Trigger_1/1 -> Switch/2
  Vector Concatenate2/1 -> Vector Concatenate1/1
  Vector Concatenate3/1 -> Switch/3, Vector Concatenate1/2
  Switch/1 -> h_k/1
  Vector Concatenate1/1 -> Switch/1

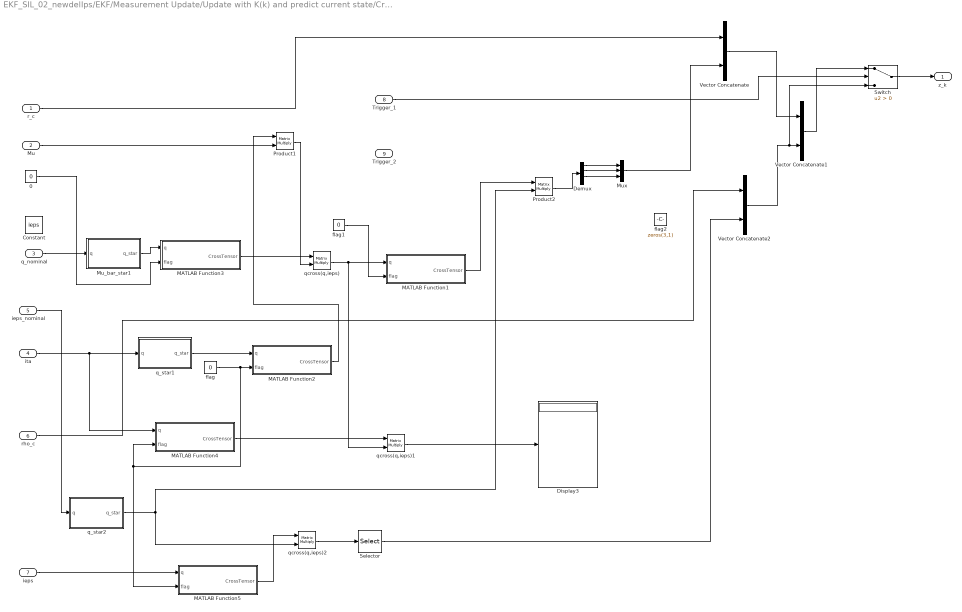
== system EKF_SIL_02_newdelIps/EKF/Measurement Update/Update with K(k) and predict current state/Create observation ==
  r_c : Inport
  Mu : Inport  Port=2
  q_nominal : Inport  Port=3
  ita : Inport  Port=4
  ieps_nominal : Inport  Port=5
  rho_c : Inport  Port=6
  ieps : Inport  Port=7
  Trigger_1 : Inport  Port=8
  Trigger_2 : Inport  Port=9
  0 : Constant  Value=0
  Constant : Constant  Value=ieps
  Demux : Demux
  Display3 : Display
  MATLAB Function1 : MATLAB Function  TreatAsAtomicUnit=on
  MATLAB Function2 : MATLAB Function  TreatAsAtomicUnit=on
  MATLAB Function3 : MATLAB Function  TreatAsAtomicUnit=on
  MATLAB Function4 : MATLAB Function  TreatAsAtomicUnit=on
  MATLAB Function5 : MATLAB Function  TreatAsAtomicUnit=on
  Mu_bar_star1 : Subsystem
  Mux : Mux  Inputs=3
  Product1 : Product  Multiplication=Matrix(*)
  Product2 : Product  Multiplication=Matrix(*)
  Selector : Selector  InputPortWidth=4  Indices=[1:3]
  Switch : Switch  Criteria=u2 > Threshold  AllowDiffInputSizes=on
  Vector Concatenate : Concatenate
  Vector Concatenate1 : Concatenate
  Vector Concatenate2 : Concatenate
  flag : Constant  Value=0
  flag1 : Constant  Value=0
  flag2 : Constant  Value=zeros(3,1)
  q_star1 : Subsystem
  q_star2 : Subsystem
  qcross(q,ieps) : Product  Multiplication=Matrix(*)
  qcross(q,ieps)1 : Product  Multiplication=Matrix(*)
  qcross(q,ieps)2 : Product  Multiplication=Matrix(*)
  z_k : Outport
  wires:
  MATLAB Function2/1(CrossTensor) -> Product1/1
  flag/1 -> MATLAB Function2/2(flag), MATLAB Function4/2(flag), MATLAB Function5/2(flag)
  q_star1/1(q_star) -> MATLAB Function2/1(q)
  ita/1 -> MATLAB Function4/1(q), q_star1/1(q)
  Demux/1 -> Mux/1
  Demux/2 -> Mux/2
  Demux/3 -> Mux/3
  Mux/1 -> Vector Concatenate/2
  0/1 -> MATLAB Function3/2(flag)
  r_c/1 -> Vector Concatenate/1
  MATLAB Function1/1(CrossTensor) -> Product2/1
  Product2/1 -> Demux/1
  q_nominal/1 -> Mu_bar_star1/1(q)
  MATLAB Function3/1(CrossTensor) -> qcross(q,ieps)/1
  ieps_nominal/1 -> q_star2/1(q)
  qcross(q,ieps)/1 -> qcross(q,ieps)1/2, MATLAB Function1/1(q)
  Mu/1 -> Product1/2
  MATLAB Function4/1(CrossTensor) -> qcross(q,ieps)1/1
  qcross(q,ieps)1/1 -> Display3/1
  flag1/1 -> MATLAB Function1/2(flag)
  rho_c/1 -> Vector Concatenate2/1
  q_star2/1(q_star) -> qcross(q,ieps)2/2, Product2/2
  MATLAB Function5/1(CrossTensor) -> qcross(q,ieps)2/1
  ieps/1 -> MATLAB Function5/1(q)
  qcross(q,ieps)2/1 -> Selector/1
  Selector/1 -> Vector Concatenate2/2
  Mu_bar_star1/1(q_star) -> MATLAB Function3/1(q)
  Product1/1 -> qcross(q,ieps)/2
  Vector Concatenate/1 -> Vector Concatenate1/1
  Trigger_1/1 -> Switch/2
  Vector Concatenate2/1 -> Switch/3, Vector Concatenate1/2
  Switch/1 -> z_k/1
  Vector Concatenate1/1 -> Switch/1

== system EKF_SIL_02_newdelIps/EKF/Measurement Update/Update with K(k) and predict current state/K*H ==
  H : Inport
  K : Inport  Port=2
  MATLAB Function : MATLAB Function  TreatAsAtomicUnit=on
  K*H : Outport
  wires:
  K/1 -> MATLAB Function/1(K)
  H/1 -> MATLAB Function/2(H)
  MATLAB Function/1(y) -> K*H/1

== system EKF_SIL_02_newdelIps/EKF/Measurement Update/Update with K(k) and predict current state/Kalman gain ==
  H_k : Inport
  P_pre : Inport  Port=2
  S_k : Inport  Port=3
  Display3 : Display
  MATLAB Function : MATLAB Function  TreatAsAtomicUnit=on
  Math Function1 : Math  Operator=log10  SaturateOnIntegerOverflow=on
  Scope : Scope
      settings: YMin=-1.61  YMax=-1.41  SaveName=ScopeData22
  Selector : Selector  NumberOfDimensions=2  InputPortWidth=3  IndexOptions=Index vector (dialog),Index vector (dialog)  Indices=[1:6],[1:6]  OutputSizes=1,1
  Sum of Elements : Sum  Inputs=+
  K : Outport
  H.P(k|k-1).H' + S_k : Outport  Port=2
  wires:
  H_k/1 -> MATLAB Function/1(H)
  P_pre/1 -> MATLAB Function/2(P_pre)
  Selector/1 -> Sum of Elements/1
  Sum of Elements/1 -> Math Function1/1
  Math Function1/1 -> Scope/1
  S_k/1 -> MATLAB Function/3(S_k)
  MATLAB Function/1(K) -> K/1
  MATLAB Function/2(Cov_x_y) -> H.P(k|k-1).H' + S_k/1, Selector/1

== system EKF_SIL_02_newdelIps/EKF/Measurement Update/Update with K(k) and predict current state/MhDist ==
  x : Inport
  Var : Inport  Port=2
  MATLAB Function : MATLAB Function  TreatAsAtomicUnit=on
  d^2 : Outport
  wires:
  MATLAB Function/1(y) -> d^2/1
  x/1 -> MATLAB Function/1(x)
  Var/1 -> MATLAB Function/2(Var)

== system EKF_SIL_02_newdelIps/EKF/Measurement Update/Update with K(k) and predict current state/Outlier rejector ==
  Computed K : Inport
  X^2 : Inport  Port=2
  Chi_threshold : Constant  Value=1000
  Relational Operator : RelationalOperator  Operator=<  OutDataTypeStr=boolean
  Scope : Scope
      settings: ShowLegends=on  SaveName=ScopeData31
  Switch : Switch  Criteria=u2 > Threshold
  zeros(12,) : Constant  Value=zeros(12,6)
  K (outlier_checked) : Outport
  wires:
  Computed K/1 -> Switch/1
  X^2/1 -> Relational Operator/1
  Chi_threshold/1 -> Relational Operator/2
  Relational Operator/1 -> Switch/2, Scope/1  "Outlier rejector (Not)"
  Switch/1 -> K (outlier_checked)/1
  zeros(12,)/1 -> Switch/3

== system EKF_SIL_02_newdelIps/EKF/Measurement Update/Update with K(k) and predict current state/Subsystem ==
  residual : Inport
  K : Inport  Port=2
  MATLAB Function : MATLAB Function  TreatAsAtomicUnit=on
  K(z-h(x)) : Outport
  wires:
  MATLAB Function/1(y) -> K(z-h(x))/1
  K/1 -> MATLAB Function/1(K)
  residual/1 -> MATLAB Function/2(del_x)

== system EKF_SIL_02_newdelIps/EKF/Predictor/Create State error covariance (P)/Process noise covariance [rotational] ==
  Phi : Inport
  Process Noise covariance : MATLAB Function  TreatAsAtomicUnit=on
  p : Constant  Value=[p_x;p_y;p_z]
  sig_tau : Constant  Value=sig_tau
  t_delta : Constant  Value=t_Kalman
  Q_r : Outport
  wires:
  Phi/1 -> Process Noise covariance/1(Phi)
  t_delta/1 -> Process Noise covariance/3(t_delta)
  sig_tau/1 -> Process Noise covariance/4(tau)
  p/1 -> Process Noise covariance/6(p)
  Process Noise covariance/1(Q_r) -> Q_r/1

== system EKF_SIL_02_newdelIps/EKF/Predictor/Create State error covariance (P)/Process noise covariance [translational] ==
  Process noise covariance [translational] : MATLAB Function  TreatAsAtomicUnit=on
  n : Constant  Value=n
  sig_f : Constant  Value=sig_f
  t_Kalman : Constant  Value=t_Kalman
  Q_t : Outport
  wires:
  n/1 -> Process noise covariance [translational]/2(n)
  t_Kalman/1 -> Process noise covariance [translational]/1(t_Kalman)
  sig_f/1 -> Process noise covariance [translational]/3(sigma_f)
  Process noise covariance [translational]/1(Q_t_k) -> Q_t/1

== system EKF_SIL_02_newdelIps/EKF/Predictor/Create State error covariance (P)/State Propagation ==
  "X_a(t)\t" : Inport
  V : Inport  Port=2
  Bus Selector : BusSelector  OutputSignals=ieps
  Create M : Subsystem
  Create Rotation Matrix 1 : Subsystem
  MATLAB Function : MATLAB Function  TreatAsAtomicUnit=on
  Math Function : Math  Operator=transpose  SaturateOnIntegerOverflow=on
  Product : Product  Multiplication=Matrix(*)
  Selector : Selector  InputPortWidth=6  Indices=[4:6]
  Signal Specification : SignalSpecification  Dimensions=[18,18]
  n : Constant  Value=n
  p : Constant  Value=[p_x;p_y;p_z]
  "t_Kalman " : Constant  Value=t_Kalman
  Phi : Outport
  wires:
  p/1 -> Create M/2(p), MATLAB Function/4(p)
  n/1 -> MATLAB Function/2(n)
  "t_Kalman "/1 -> MATLAB Function/3(t_Kalman)
  MATLAB Function/1(Phi) -> Signal Specification/1
  "X_a(t)\t"/1 -> Bus Selector/1, Create M/1("X_a "), MATLAB Function/1(X_a)
  Create M/1(M) -> MATLAB Function/5(M)
  V/1 -> Selector/1, MATLAB Function/6(V)
  Signal Specification/1 -> Phi/1
  Bus Selector/1 -> Create Rotation Matrix 1/1(q)  "<ieps>"
  Create Rotation Matrix 1/1(R) -> Math Function/1
  Selector/1 -> Product/2
  Product/1 -> MATLAB Function/7(om_EE)
  Math Function/1 -> Product/1

== system EKF_SIL_02_newdelIps/EKF/Predictor/Dynamic Model (Differential equations)2/Dynamic Model (Differential equations) ==
  X_a(t) : Inport
  "V " : Inport  Port=2
  Bus Creator : BusCreator  Inputs=6
  Constant : Constant  Value=[0]  SampleTime=-1
  Constant1 : Constant  Value=zeros(3,1)
  "Orbital Dynamics " : Subsystem
  Pose Servicer base/EE : Subsystem
  Quaternion Kinematics : Subsystem
  Rotational Dynamics : Subsystem
  Vector Concatenate : Concatenate
  ieps : Selector  NumberOfDimensions=2  InputPortWidth=3  IndexOptions=Index vector (dialog),Index vector (dialog)  Indices=[17:20],1  OutputSizes=1,1
  n : Constant  Value=n  SampleTime=-1
  omega : Selector  NumberOfDimensions=2  InputPortWidth=3  IndexOptions=Index vector (dialog),Index vector (dialog)  Indices=[5 6 7],1  OutputSizes=1,1
  p : Constant  Value=[p_x;p_y;p_z]  SampleTime=-1
  parameter_gravitation : Constant  Value=parameter_gravitation  SampleTime=-1
  q : Selector  NumberOfDimensions=2  InputPortWidth=3  IndexOptions=Index vector (dialog),Index vector (dialog)  Indices=[1 2 3 4],1  OutputSizes=1,1
  r : Selector  NumberOfDimensions=2  InputPortWidth=3  IndexOptions=Index vector (dialog),Index vector (dialog)  Indices=[8 9 10],1  OutputSizes=1,1
  r_dot : Selector  NumberOfDimensions=2  InputPortWidth=3  IndexOptions=Index vector (dialog),Index vector (dialog)  Indices=[11 12 13],1  OutputSizes=1,1
  rho_c : Selector  NumberOfDimensions=2  InputPortWidth=3  IndexOptions=Index vector (dialog),Index vector (dialog)  Indices=[14 15 16],1  OutputSizes=1,1
  X_a(t+1) : Outport
  wires:
  Bus Creator/1 -> X_a(t+1)/1
  r_dot/1 -> Bus Creator/3, "Orbital Dynamics "/4("r_dot ")
  r/1 -> "Orbital Dynamics "/1(r)
  omega/1 -> Vector Concatenate/1, Rotational Dynamics/1(omega)
  q/1 -> Quaternion Kinematics/1(q)
  X_a(t)/1 -> r/1, ieps/1, rho_c/1, r_dot/1, omega/1, q/1
  Rotational Dynamics/1(omega_dot) -> Bus Creator/2  "omega_dot"
  Quaternion Kinematics/1(q_dot) -> Bus Creator/1  "q_dot"
  Constant1/1 -> Bus Creator/4  "r_ddot"
  n/1 -> "Orbital Dynamics "/3(n)
  parameter_gravitation/1 -> "Orbital Dynamics "/2(Mu)
  Vector Concatenate/1 -> Quaternion Kinematics/2(omega_rel)
  p/1 -> Rotational Dynamics/2(p)
  Constant/1 -> Vector Concatenate/2
  Pose Servicer base/EE/1(rho_c_dot) -> Bus Creator/5  "rho_c_dot"
  Pose Servicer base/EE/2(ieps_dot) -> Bus Creator/6  "ieps_dot"
  "V "/1 -> Pose Servicer base/EE/1(V)
  rho_c/1 -> Pose Servicer base/EE/2(rho_c)
  ieps/1 -> Pose Servicer base/EE/3("ieps ")

== system EKF_SIL_02_newdelIps/Plant/Dynamic Model (Differential equations)/Orbital Dynamics /Create Skew Symmetric ==
  vector : Inport
  0 : Constant  Value=0
  Create 3x3 matrix : Subsystem
  Demux : Demux  Outputs=3
  Demux1 : Demux  Outputs=3
  Gain : Gain  Gain=-1
  skew symmetric Matrix : Outport
  wires:
  0/1 -> Create 3x3 matrix/1(a11), Create 3x3 matrix/5(a22), Create 3x3 matrix/9(a33)
  Demux/3 -> Create 3x3 matrix/2(a12)
  Demux1/2 -> Create 3x3 matrix/3(a13)
  Demux1/3 -> Create 3x3 matrix/4(a21)
  Demux/1 -> Create 3x3 matrix/6(a23)
  vector/1 -> Demux1/1, Gain/1
  Create 3x3 matrix/1(Matrix) -> skew symmetric Matrix/1
  Gain/1 -> Demux/1
  Demux/2 -> Create 3x3 matrix/7(a31)
  Demux1/1 -> Create 3x3 matrix/8(a32)

== system EKF_SIL_02_newdelIps/Plant/Dynamic Model (Differential equations)/Orbital Dynamics /norm  ==
  vector : Inport
  Dot Product : DotProduct  InputSameDT=on  OutDataTypeStr=Inherit: Inherit via internal rule
  Sqrt : Sqrt  SaturateOnIntegerOverflow=on
  "norm " : Outport
  wires:
  Dot Product/1 -> Sqrt/1
  vector/1 -> Dot Product/2, Dot Product/1
  Sqrt/1 -> "norm "/1

== system EKF_SIL_02_newdelIps/Plant/Dynamic Model (Differential equations)/Rotational Dynamics/Create  J ==
  p : Inport
  0 : Constant  Value=0
  1 : Constant
  Create 3x3 matrix : Subsystem
  Fcn : Fcn  Expr=1-u(2)/1+u(1)
  Fcn1 : Fcn  Expr=1+u(3)/1-u(1)
  "J_k " : Outport
  wires:
  Fcn/1 -> Create 3x3 matrix/5(a22)
  p/1 -> Fcn1/1, Fcn/1
  0/1 -> Create 3x3 matrix/2(a12), Create 3x3 matrix/3(a13), Create 3x3 matrix/4(a21), Create 3x3 matrix/6(a23), Create 3x3 matrix/7(a31), Create 3x3 matrix/8(a32)
  Create 3x3 matrix/1(Matrix) -> "J_k "/1
  Fcn1/1 -> Create 3x3 matrix/9(a33)
  1/1 -> Create 3x3 matrix/1(a11)

== system EKF_SIL_02_newdelIps/Plant/Dynamic Model (Differential equations)/Rotational Dynamics/Create Psi ==
  "omega " : Inport
  p : Inport  Port=2
  Create Psi : Concatenate  NumInputs=3
  Demux : Demux  Outputs=3
  Demux1 : Demux  Outputs=3
  Product{,1..5} (6 alike) : Product
  Psi : Outport
  wires:
  Demux1/3 -> Product1/2, Product3/2
  p/1 -> Demux/1
  Demux/3 -> Product4/1
  Product4/1 -> Create Psi/3
  Demux1/1 -> Product5/2, Product3/1
  Demux1/2 -> Product1/1, Product5/1
  Product2/1 -> Create Psi/2
  Demux/1 -> Product/1
  Create Psi/1 -> Psi/1
  Demux/2 -> Product2/1
  Product/1 -> Create Psi/1
  Product1/1 -> Product/2
  Product5/1 -> Product4/2
  Product3/1 -> Product2/2
  "omega "/1 -> Demux1/1

== system EKF_SIL_02_newdelIps/Plots and display/Create Measurements [Pose]1/Create Measurements [Position]/Create Rotation Matrix  ==
  q : Inport
  Add : Sum
  Add5 : Sum  Inputs=+++
  Constant1 : Constant  Value=-1
  Create Skew Symmetric : Subsystem
  Gain : Gain  Gain=2
  Gain1 : Gain  Gain=2
  Gain2 : Gain  Gain=2
  I : Constant  Value=eye(3,3)
  Math Function : Math  Operator=square  SaturateOnIntegerOverflow=on
  Math Function1 : Math  Operator=transpose  SaturateOnIntegerOverflow=on
  Product1 : Product
  Product2 : Product
  Product3 : Product  Multiplication=Matrix(*)
  Selector2 : Selector  NumberOfDimensions=2  InputPortWidth=3  IndexOptions=Index vector (dialog),Index vector (dialog)  Indices=[1 2 3],1  OutputSizes=1,1
  Selector3 : Selector  NumberOfDimensions=2  InputPortWidth=3  IndexOptions=Index vector (dialog),Index vector (dialog)  Indices=[4],1  OutputSizes=1,1
  R : Outport
  wires:
  q/1 -> Selector2/1, Selector3/1
  Add5/1 -> R/1
  Product3/1 -> Gain2/1
  Math Function1/1 -> Product3/2
  Product1/1 -> Add5/3
  Gain1/1 -> Product2/1
  Create Skew Symmetric/1(skew symmetric Matrix) -> Gain1/1
  Product2/1 -> Add5/2
  Gain2/1 -> Add5/1
  Selector2/1 -> Create Skew Symmetric/1(vector), Product3/1, Math Function1/1
  I/1 -> Product1/2
  Add/1 -> Product1/1
  Selector3/1 -> Math Function/1, Product2/2
  Constant1/1 -> Add/2
  Math Function/1 -> Gain/1
  Gain/1 -> Add/1

== system EKF_SIL_02_newdelIps/Plots and display/Create Measurements [Pose]2/Create Measurements [Position]/Create Rotation Matrix  ==
  q : Inport
  Add : Sum
  Add5 : Sum  Inputs=+++
  Constant1 : Constant  Value=-1
  Create Skew Symmetric : Subsystem
  Gain : Gain  Gain=2
  Gain1 : Gain  Gain=2
  Gain2 : Gain  Gain=2
  I : Constant  Value=eye(3,3)
  Math Function : Math  Operator=square  SaturateOnIntegerOverflow=on
  Math Function1 : Math  Operator=transpose  SaturateOnIntegerOverflow=on
  Product1 : Product
  Product2 : Product
  Product3 : Product  Multiplication=Matrix(*)
  Selector2 : Selector  NumberOfDimensions=2  InputPortWidth=3  IndexOptions=Index vector (dialog),Index vector (dialog)  Indices=[1 2 3],1  OutputSizes=1,1
  Selector3 : Selector  NumberOfDimensions=2  InputPortWidth=3  IndexOptions=Index vector (dialog),Index vector (dialog)  Indices=[4],1  OutputSizes=1,1
  R : Outport
  wires:
  Gain/1 -> Add/1
  Math Function/1 -> Gain/1
  Constant1/1 -> Add/2
  Selector3/1 -> Product2/2, Math Function/1
  Add/1 -> Product1/1
  I/1 -> Product1/2
  Selector2/1 -> Math Function1/1, Product3/1, Create Skew Symmetric/1(vector)
  Gain2/1 -> Add5/1
  Product2/1 -> Add5/2
  Create Skew Symmetric/1(skew symmetric Matrix) -> Gain1/1
  Gain1/1 -> Product2/1
  Product1/1 -> Add5/3
  Math Function1/1 -> Product3/2
  Product3/1 -> Gain2/1
  Add5/1 -> R/1
  q/1 -> Selector3/1, Selector2/1
